simulink model "Part2_III"  (R2023b)
settings: Solver=VariableStepAuto  StartTime=0.0  StopTime=1  RelTol=1e-3
libraries: commrandsrc3 x1, commfilt2 x1
settings Model: Creator=henry  LastModifiedBy=henry

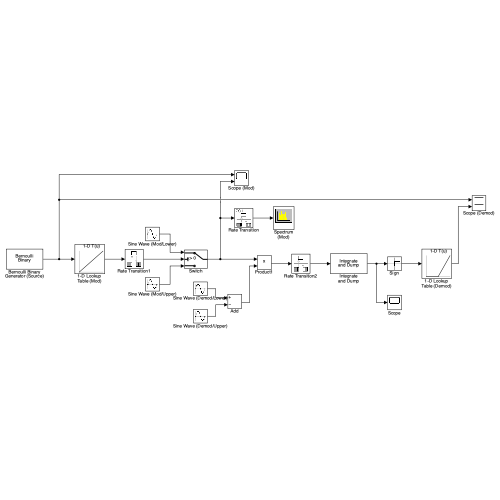
[thumbnail: Simulink's stored preview of the top-level diagram]
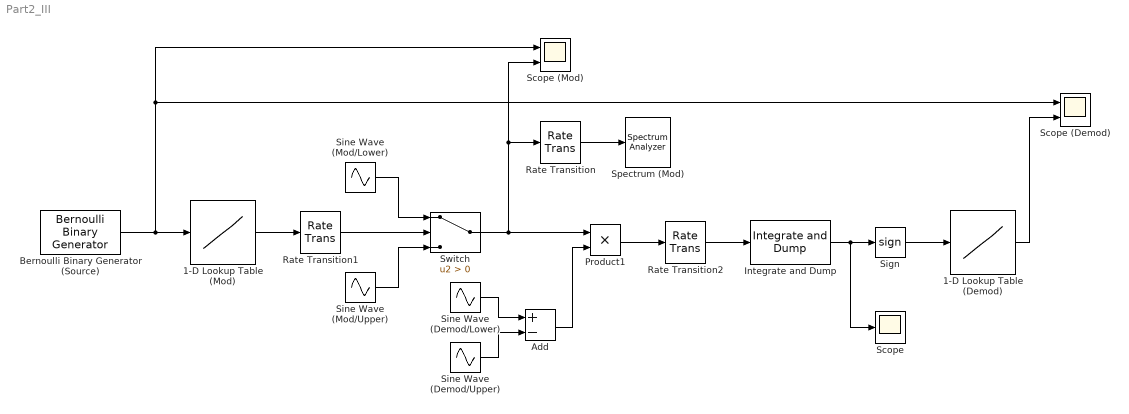
== system Part2_III ==
  1-D Lookup Table (Demod) : Lookup_n-D  NumberOfTableDimensions=1  BreakpointsForDimension1=[-1,0,1]  Table=[0,0,1]  InternalRulePriority=Speed  RndMeth=Simplest
  1-D Lookup Table (Mod) : Lookup_n-D  NumberOfTableDimensions=1  BreakpointsForDimension1=[0,1]  Table=[-1,1]  InternalRulePriority=Speed  RndMeth=Simplest
  Add : Sum  Inputs=+-
  Bernoulli Binary Generator (Source) : commrandsrc3/Bernoulli Binary Generator  ProbabilityOfZero=0.5  SeedSource=Parameter  Seed=100  SampleTime=0.001  SamplesPerFrame=1  OutputDataType=double  SimulateUsing=Interpreted execution
  Integrate and Dump : commfilt2/Integrate and Dump  obssamples=8  offsetsamples=0  nodump=off  roundingMode=Floor  overflowMode=off  outputDataTypeStr=Inherit: Same as accumulator  outputLastDataTypeStr=Inherit: Same as accumulator
  Product1 : Product
  Rate Transition : RateTransition  OutPortSampleTime=0.5e-4
  Rate Transition1 : RateTransition  OutPortSampleTime=0.5e-4
  Rate Transition2 : RateTransition  OutPortSampleTime=0.5e-4
  Scope : Scope
  Scope (Demod) : Scope  NumInputPorts=2
  Scope (Mod) : Scope  NumInputPorts=2
  Sign : Signum
  Sine Wave (Demod/Lower) : Sin  SineType=Sample based  Samples=4000  SampleTime=1e-7
  Sine Wave (Demod/Upper) : Sin  SineType=Sample based  Samples=2857  SampleTime=1e-7
  Sine Wave (Mod/Lower) : Sin  SineType=Sample based  Samples=4000  SampleTime=1e-7
  Sine Wave (Mod/Upper) : Sin  SineType=Sample based  Samples=2857  SampleTime=1e-7
  Spectrum (Mod) : SpectrumAnalyzer  WindowPosition=[320.000000,200.000000,800.000000,500.000000,]  ScopeFrameLocation=window  Span=20000  StartFrequency=-10000  StopFrequency=10000  YLimits=[-64.5412526,26.44952389]
  Switch : Switch  Criteria=u2 > Threshold  SaturateOnIntegerOverflow=off  InputSameDT=off
  wires:
  Bernoulli Binary Generator (Source)/1 -> Scope (Demod)/1, Scope (Mod)/1, 1-D Lookup Table (Mod)/1
  1-D Lookup Table (Mod)/1 -> Rate Transition1/1
  Rate Transition1/1 -> Switch/2
  Sine Wave (Mod/Lower)/1 -> Switch/1
  Sine Wave (Mod/Upper)/1 -> Switch/3
  Sine Wave (Demod/Lower)/1 -> Add/1
  Sine Wave (Demod/Upper)/1 -> Add/2
  Switch/1 -> Rate Transition/1, Scope (Mod)/2, Product1/1
  Add/1 -> Product1/2
  Product1/1 -> Rate Transition2/1
  Rate Transition2/1 -> Integrate and Dump/1
  Integrate and Dump/1 -> Scope/1, Sign/1
  Sign/1 -> 1-D Lookup Table (Demod)/1
  Rate Transition/1 -> Spectrum (Mod)/1
  1-D Lookup Table (Demod)/1 -> Scope (Demod)/2
